simulink model "EPD629_WilliamsJ_AS02_simulink"  (R2021b)
settings: Solver=VariableStepAuto  StartTime=0.0  StopTime=2000  RelTol=1e-3
values from neighbouring files (symbols this model uses):
  AeroArea_m2 = 10    [AS02.m]    (also in EPD629_WilliamsJ_AS02.m)
  AeroDragCoef = 0.6    [AS02.m]    (also in EPD629_WilliamsJ_AS02.m)
  AirGasConstant_kJpkgK = 0.278    [AS02.m]    (also in EPD629_WilliamsJ_AS02.m)
  AmbientPress_kPa = 100    [AS02.m]    (also in EPD629_WilliamsJ_AS02.m)
  AmbientTemp_C = 20    [AS02.m]    (also in EPD629_WilliamsJ_AS02.m)
  CelsiusToKelvinConstant = 273.15    [AS02.m]    (also in EPD629_WilliamsJ_AS02.m)
  GravitationalAccel_mps2 = 9.8067    [AS02.m]    (also in EPD629_WilliamsJ_AS02.m)
  PitchAngleData_deg = [2 2]    [AS02.m]    (also in EPD629_WilliamsJ_AS02.m)
  PitchAnglePositionBP_m = [0 1e6]    [AS02.m]    (also in EPD629_WilliamsJ_AS02.m)
  RollingDragCoef = 0.005    [AS02.m]    (also in EPD629_WilliamsJ_AS02.m)
  VehicleMass_kg = 30000    [AS02.m]    (also in EPD629_WilliamsJ_AS02.m)
settings Model: Creator=jwilli42  LastModifiedBy=jwilli42

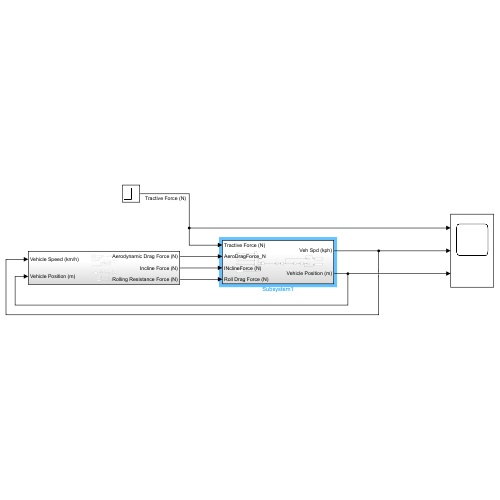
[thumbnail: Simulink's stored preview of the top-level diagram]
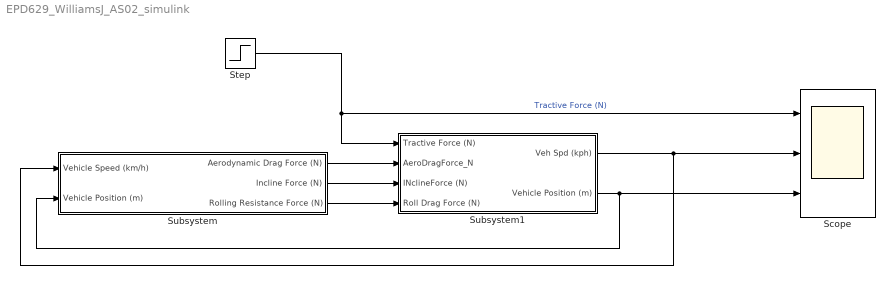
== system EPD629_WilliamsJ_AS02_simulink ==
  Scope : Scope  NumInputPorts=3
  Step : Step  Time=1000  Before=13000  After=15000  SampleTime=0
  Subsystem : Subsystem
  Subsystem1 : Subsystem
  wires:
  Subsystem1/1(Veh Spd (kph)) -> Scope/2, Subsystem/1(Vehicle Speed (km/h))
  Subsystem1/2(Vehicle Position (m)) -> Subsystem/2(Vehicle Position (m)), Scope/3
  Subsystem/3(Rolling Resistance Force (N)) -> Subsystem1/4(Roll Drag Force (N))
  Step/1 -> Scope/1, Subsystem1/1(Tractive Force (N))  "Tractive Force (N)"
  Subsystem/1(Aerodynamic Drag Force (N)) -> Subsystem1/2(AeroDragForce_N)
  Subsystem/2(Incline Force (N)) -> Subsystem1/3(INclineForce (N))

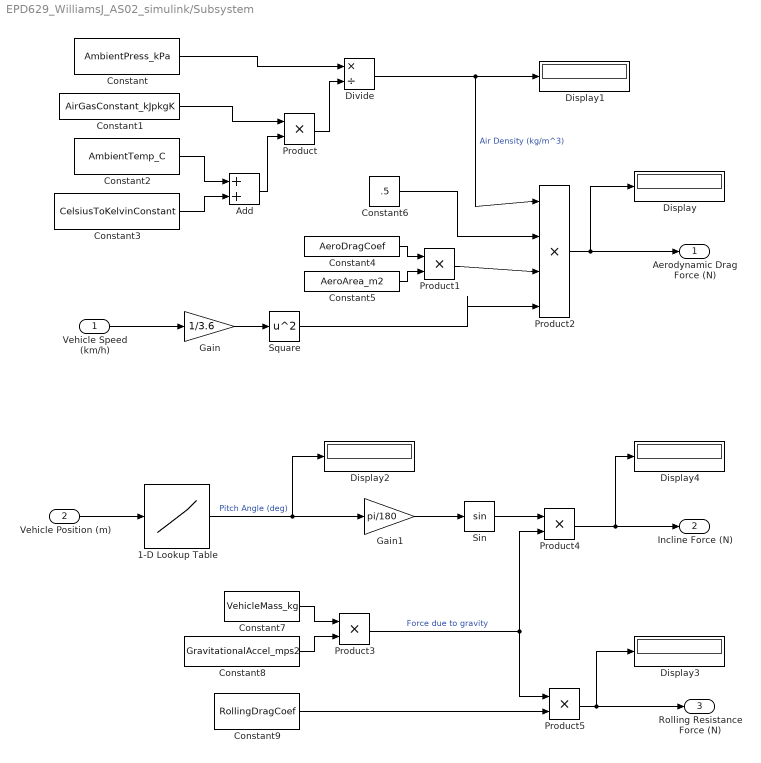
== system EPD629_WilliamsJ_AS02_simulink/Subsystem ==
  Vehicle Speed (km/h) : Inport
  Vehicle Position (m) : Inport  Port=2
  1-D Lookup Table : Lookup_n-D  NumberOfTableDimensions=1  BreakpointsForDimension1=PitchAnglePositionBP_m  Table=PitchAngleData_deg  ExtrapMethod=Clip  UseLastTableValue=on  InternalRulePriority=Speed  RndMeth=Simplest  InputSameDT=on
  Add : Sum
  Constant : Constant  Value=AmbientPress_kPa
  Constant1 : Constant  Value=AirGasConstant_kJpkgK
  Constant2 : Constant  Value=AmbientTemp_C
  Constant3 : Constant  Value=CelsiusToKelvinConstant
  Constant4 : Constant  Value=AeroDragCoef
  Constant5 : Constant  Value=AeroArea_m2
  Constant6 : Constant  Value=.5
  Constant7 : Constant  Value=VehicleMass_kg
  Constant8 : Constant  Value=GravitationalAccel_mps2
  Constant9 : Constant  Value=RollingDragCoef
  Display{,1..4} (5 alike) : Display
  Divide : Product  Inputs=*/
  Gain : Gain  Gain=1/3.6
  Gain1 : Gain  Gain=pi/180
  Product{,1,3..5} (5 alike) : Product
  Product2 : Product  Inputs=4
  Sin : Trigonometry
  Square : Math  Operator=square  SaturateOnIntegerOverflow=on
  Aerodynamic Drag Force (N) : Outport
  Incline Force (N) : Outport  Port=2
  Rolling Resistance Force (N) : Outport  Port=3
  wires:
  Product4/1 -> Incline Force (N)/1, Display4/1
  Constant/1 -> Divide/1
  Gain1/1 -> Sin/1
  Product2/1 -> Aerodynamic Drag Force (N)/1, Display/1
  Constant3/1 -> Add/2
  Product5/1 -> Rolling Resistance Force (N)/1, Display3/1
  Constant2/1 -> Add/1
  Product3/1 -> Product5/1, Product4/2  "Force due to gravity"
  Constant7/1 -> Product3/1
  Gain/1 -> Square/1
  Divide/1 -> Product2/1, Display1/1  "Air Density (kg/m^3)"
  1-D Lookup Table/1 -> Display2/1, Gain1/1  "Pitch Angle (deg)"
  Vehicle Position (m)/1 -> 1-D Lookup Table/1
  Product/1 -> Divide/2
  Constant1/1 -> Product/1
  Add/1 -> Product/2
  Product1/1 -> Product2/3
  Square/1 -> Product2/4
  Constant4/1 -> Product1/1
  Constant5/1 -> Product1/2
  Vehicle Speed (km/h)/1 -> Gain/1
  Constant6/1 -> Product2/2
  Constant8/1 -> Product3/2
  Constant9/1 -> Product5/2
  Sin/1 -> Product4/1

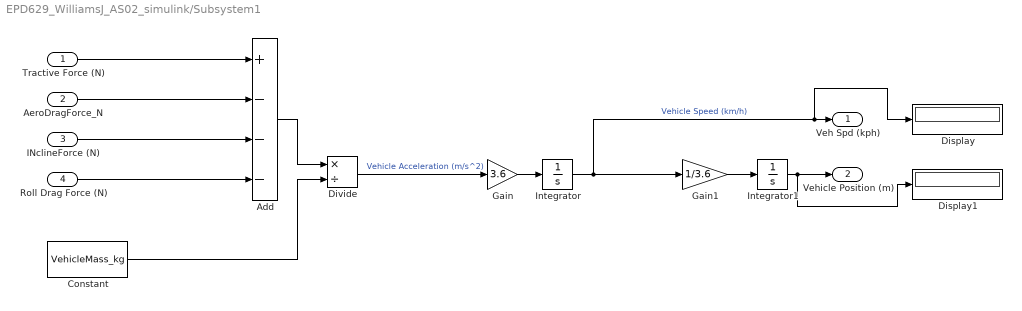
== system EPD629_WilliamsJ_AS02_simulink/Subsystem1 ==
  Tractive Force (N) : Inport
  AeroDragForce_N : Inport  Port=2
  INclineForce (N) : Inport  Port=3
  Roll Drag Force (N) : Inport  Port=4
  Add : Sum  Inputs=+---
  Constant : Constant  Value=VehicleMass_kg
  Display : Display
  Display1 : Display
  Divide : Product  Inputs=*/
  Gain : Gain  Gain=3.6
  Gain1 : Gain  Gain=1/3.6
  Integrator : Integrator  LimitOutput=on  UpperSaturationLimit=150  LowerSaturationLimit=0
  Integrator1 : Integrator  LimitOutput=on  UpperSaturationLimit=1e6  LowerSaturationLimit=0
  Veh Spd (kph) : Outport
  Vehicle Position (m) : Outport  Port=2
  wires:
  Gain/1 -> Integrator/1
  AeroDragForce_N/1 -> Add/2
  Roll Drag Force (N)/1 -> Add/4
  Integrator1/1 -> Vehicle Position (m)/1, Display1/1
  Divide/1 -> Gain/1  "Vehicle Acceleration (m/s^2)"
  INclineForce (N)/1 -> Add/3
  Integrator/1 -> Display/1, Veh Spd (kph)/1, Gain1/1  "Vehicle Speed (km/h)"
  Gain1/1 -> Integrator1/1
  Constant/1 -> Divide/2
  Tractive Force (N)/1 -> Add/1
  Add/1 -> Divide/1
